simulink model "demo_gs1"  (Simulink 2.20)
settings: Solver=ode45  StartTime=0.0  StopTime=30  MaxStep=0.1  RelTol=1e-3  AbsTol=1e-6
values from neighbouring files (symbols this model uses):
  x1 = x(j)    [fazrov_auton2.m]
  x2 = x(j+1)    [fazrov_auton2.m]    (also in fazrov_typ1.m = get_param(get_param(gcbh,'Parent'),'UserData'))
undefined symbols (not defined in the file or in its folder): w
libraries: NelinSys x4
settings Model: ConsistencyChecking=off  RTWPlaceOutputsASAP=off

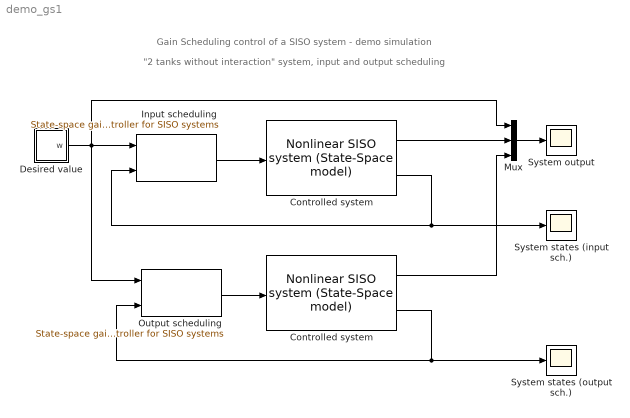
== system demo_gs1 ==
  note: Gain Scheduling control of a SISO system - demo simulation
  note: "2 tanks without interaction" system, input and output scheduling
  " Controlled system " : NelinSys/Nonlinear Systems Synthesis/Nonlinear SISO system (State-Space model)  n=2  F=[-sqrt(x1); sqrt(x1)-sqrt(x2)]  Fp=0  G=[1; 0]  Gp=0  H=x2  Hp=0  pp=[0.1; 0.01]
  Controlled system : NelinSys/Nonlinear Systems Synthesis/Nonlinear SISO system (State-Space model)  n=2  F=[-sqrt(x1); sqrt(x1)-sqrt(x2)]  Fp=0  G=[1; 0]  Gp=0  H=x2  Hp=0  pp=[0.1; 0.01]
  "Desired value " : Subsystem
  Input scheduling : NelinSys/Nonlinear Systems Synthesis/Gain Scheduling Blocks/State-space gain-scheduling controller for SISO systems  n=2  vzorec=-(-w^(1/2)+4*w)/w*x1+4*w+1/2*(-w^(1/2)+8*w-16*w^(3/2))/w*(x2-w)  vzorecP=0
  Mux : Mux  Inputs=3
  Output scheduling : NelinSys/Nonlinear Systems Synthesis/Gain Scheduling Blocks/State-space gain-scheduling controller for SISO systems  n=2  vzorec=-(-x2^(1/2)+4*x2)/x2*x1+8*x2^(1/2)*(w-x2)+4*x2  vzorecP=0
  System output : Scope
      settings: TickLabels=on  TimeRange=30  YMin=0  YMax=5  SaveToWorkspace=off  SaveName=ScopeData
  System states (input sch.) : Scope
      settings: TickLabels=on  TimeRange=30  YMin=0  YMax=8  SaveToWorkspace=off  SaveName=ScopeData
  System states (output sch.) : Scope
      settings: TickLabels=on  TimeRange=30  YMin=0  YMax=8  SaveToWorkspace=off  SaveName=ScopeData
  wires:
  Mux/1 -> System output/1
  "Desired value "/1(w) -> Mux/1, Input scheduling/1, Output scheduling/1
  Controlled system/1 -> Mux/2
  Input scheduling/1 -> Controlled system/1
  Controlled system/2 -> System states (input sch.)/1, Input scheduling/2
  Output scheduling/1 -> " Controlled system "/1
  " Controlled system "/1 -> Mux/3
  " Controlled system "/2 -> Output scheduling/2, System states (output sch.)/1

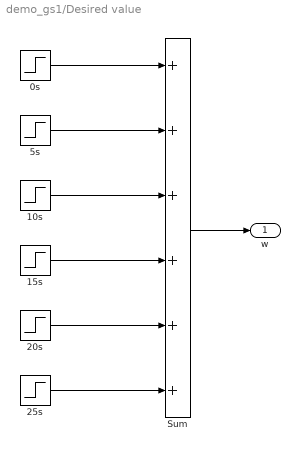
== system demo_gs1/Desired value  ==
  0s : Step  Time=0  Before=0  After=1
  10s : Step  Time=10  Before=0  After=1
  15s : Step  Time=15  Before=0  After=1
  20s : Step  Time=20  Before=0  After=1
  25s : Step  Time=25  Before=0  After=-1
  5s : Step  Time=5  Before=0  After=1
  Sum : Sum  Inputs=++++++
  w : Outport  Port=1
  wires:
  Sum/1 -> w/1
  25s/1 -> Sum/6
  20s/1 -> Sum/5
  15s/1 -> Sum/4
  10s/1 -> Sum/3
  5s/1 -> Sum/2
  0s/1 -> Sum/1
